simulink model "fahrenheitConverter_KellenHassel"  (R2025b)
settings: Solver=VariableStepAuto  StartTime=0.0  StopTime=10.0  RelTol=1e-3

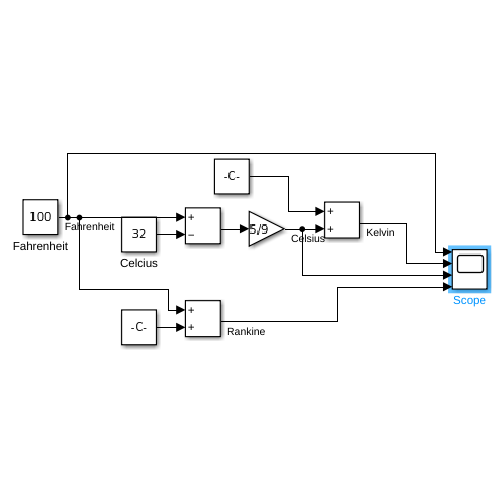
[thumbnail: Simulink's stored preview of the top-level diagram]
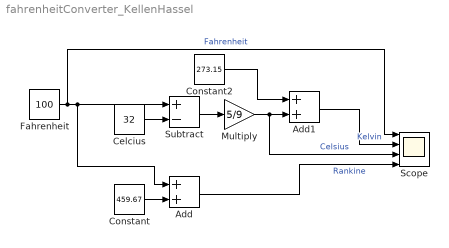
== system fahrenheitConverter_KellenHassel ==
  Add : Sum
  Add1 : Sum
  Celcius : Constant  Value=32
  Constant : Constant  Value=459.67
  Constant2 : Constant  Value=273.15
  Fahrenheit : Constant  Value=100
  Multiply : Gain  Gain=5/9
  Scope : Scope  NumInputPorts=4
      settings: ActiveDisplayYMinimum=-1014.9507057771345  ActiveDisplayYMaximum=864.71377466808292  YLabel=Temperature (°)
  Subtract : Sum  Inputs=+-
  wires:
  Fahrenheit/1 -> Scope/1, Add/1, Subtract/1  "Fahrenheit"
  Celcius/1 -> Subtract/2
  Subtract/1 -> Multiply/1
  Multiply/1 -> Scope/3, Add1/2  "Celsius"
  Constant2/1 -> Add1/1
  Constant/1 -> Add/2
  Add1/1 -> Scope/2  "Kelvin"
  Add/1 -> Scope/4  "Rankine"
